simulink library "INT_Rail_PreCtlMeUn"  (R2016b)
settings: Solver=VariableStepAuto  StartTime=0.0  StopTime=10.0  RelTol=1e-3
settings Model: Creator=mayongchao  LastModifiedBy=mayongchao

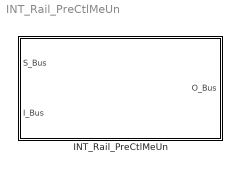
== system INT_Rail_PreCtlMeUn ==
  INT_Rail_PreCtlMeUn : Subsystem

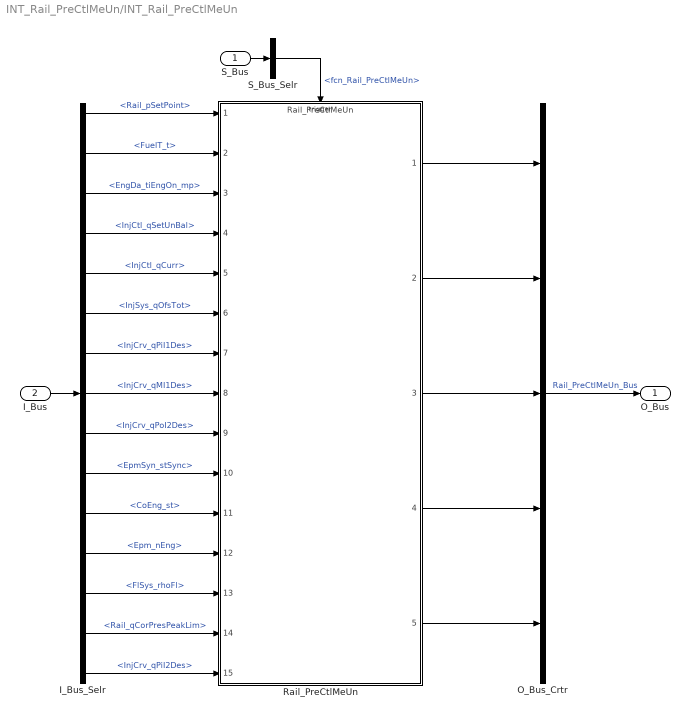
== system INT_Rail_PreCtlMeUn/INT_Rail_PreCtlMeUn ==
  S_Bus : Inport
  I_Bus : Inport  Port=2
  I_Bus_Selr : BusSelector  OutputSignals=Rail_pSetPoint,FuelT_t,EngDa_tiEngOn_mp,InjCtl_qSetUnBal,InjCtl_qCurr,InjSys_qOfsTot,InjCrv_qPiI1Des,InjCrv_qMI1Des,InjCrv_qPoI2Des,EpmSyn_stSync,CoEng_st,Epm_nEng,FlSys_rhoFl,Rail_qCorPresPeakLim,InjCrv_qPiI2Des
  O_Bus_Crtr : BusCreator  Inputs=5
  Rail_PreCtlMeUn : ModelReference  ModelNameDialog=Rail_PreCtlMeUn  SimulationMode=Normal  ModelReferenceVersion=1.60  TriggerPortName=function  TriggerPortTriggerType=function-call  TriggerPortStatesWhenEnabling=held
  S_Bus_Selr : BusSelector  OutputSignals=fcn_Rail_PreCtlMeUn
  O_Bus : Outport
  wires:
  S_Bus_Selr/1 -> Rail_PreCtlMeUn/Trigger  "<fcn_Rail_PreCtlMeUn>"
  S_Bus/1 -> S_Bus_Selr/1
  I_Bus/1 -> I_Bus_Selr/1
  I_Bus_Selr/1 -> Rail_PreCtlMeUn/1  "<Rail_pSetPoint>"
  I_Bus_Selr/2 -> Rail_PreCtlMeUn/2  "<FuelT_t>"
  I_Bus_Selr/3 -> Rail_PreCtlMeUn/3  "<EngDa_tiEngOn_mp>"
  I_Bus_Selr/4 -> Rail_PreCtlMeUn/4  "<InjCtl_qSetUnBal>"
  I_Bus_Selr/5 -> Rail_PreCtlMeUn/5  "<InjCtl_qCurr>"
  I_Bus_Selr/6 -> Rail_PreCtlMeUn/6  "<InjSys_qOfsTot>"
  I_Bus_Selr/7 -> Rail_PreCtlMeUn/7  "<InjCrv_qPiI1Des>"
  I_Bus_Selr/8 -> Rail_PreCtlMeUn/8  "<InjCrv_qMI1Des>"
  I_Bus_Selr/9 -> Rail_PreCtlMeUn/9  "<InjCrv_qPoI2Des>"
  I_Bus_Selr/10 -> Rail_PreCtlMeUn/10  "<EpmSyn_stSync>"
  I_Bus_Selr/11 -> Rail_PreCtlMeUn/11  "<CoEng_st>"
  I_Bus_Selr/12 -> Rail_PreCtlMeUn/12  "<Epm_nEng>"
  I_Bus_Selr/13 -> Rail_PreCtlMeUn/13  "<FlSys_rhoFl>"
  I_Bus_Selr/14 -> Rail_PreCtlMeUn/14  "<Rail_qCorPresPeakLim>"
  I_Bus_Selr/15 -> Rail_PreCtlMeUn/15  "<InjCrv_qPiI2Des>"
  O_Bus_Crtr/1 -> O_Bus/1  "Rail_PreCtlMeUn_Bus"
  Rail_PreCtlMeUn/1 -> O_Bus_Crtr/1
  Rail_PreCtlMeUn/2 -> O_Bus_Crtr/2
  Rail_PreCtlMeUn/3 -> O_Bus_Crtr/3
  Rail_PreCtlMeUn/4 -> O_Bus_Crtr/4
  Rail_PreCtlMeUn/5 -> O_Bus_Crtr/5
